simulink model "CPCS_nonlinear_modal"  (R2021a)
settings: Solver=VariableStepAuto  StartTime=0.0  StopTime=10.0  MaxStep=1e-4  RelTol=1e-3
values from neighbouring files (symbols this model uses):
  g = 9.81    [CPCS.m]
  M = m1+m2    (= 3.5)    [CPCS.m]
  m2 = .5    (= 0.5)    [CPCS.m]
  r = 0.5    [CPCS.m]
settings Model: Creator=raitaimoorali  LastModifiedBy=raitaimoorali

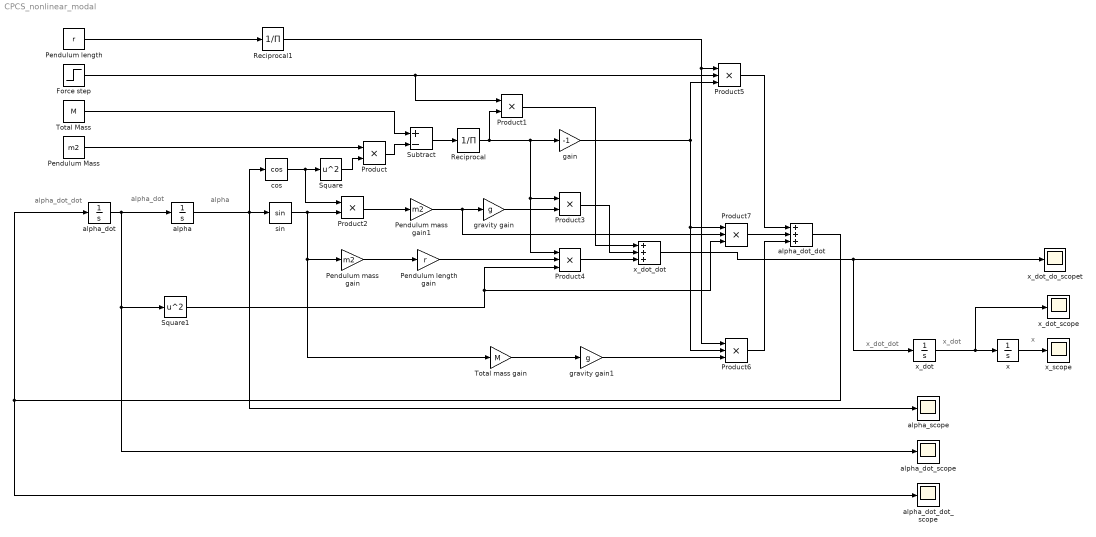
== system CPCS_nonlinear_modal ==
  note: x_dot_dot
  note: x_dot
  note: x
  note: alpha
  note: alpha_dot
  note: alpha_dot_dot
  Force step : Step  Time=0.01  SampleTime=0
  Pendulum Mass : Constant  Value=m2
  Pendulum length : Constant  Value=r
  Pendulum length gain : Gain  Gain=r
  Pendulum mass gain : Gain  Gain=m2
  Pendulum mass gain1 : Gain  Gain=m2
  Product{,1..3} (4 alike) : Product
  Product{4..7} (4 alike) : Product  Inputs=3
  Reciprocal : Product  Inputs=/
  Reciprocal1 : Product  Inputs=/
  Square : Math  Operator=square  SaturateOnIntegerOverflow=on
  Square1 : Math  Operator=square  SaturateOnIntegerOverflow=on
  Subtract : Sum  Inputs=+-
  Total Mass : Constant  Value=M
  Total mass gain : Gain  Gain=M
  alpha : Integrator
  alpha_dot : Integrator
  alpha_dot_dot : Sum  Inputs=+++
  alpha_dot_dot_scope : Scope
  alpha_dot_scope : Scope
  alpha_scope : Scope
  cos : Trigonometry  Operator=cos
  gain : Gain  Gain=-1
  gravity gain : Gain  Gain=g
  gravity gain1 : Gain  Gain=g
  sin : Trigonometry
  x : Integrator
  x_dot : Integrator
  x_dot_do_scopet : Scope
  x_dot_dot : Sum  Inputs=+++
  x_dot_scope : Scope
  x_scope : Scope
  wires:
  cos/1 -> Square/1, Product2/1
  Square/1 -> Product/2
  Pendulum Mass/1 -> Product/1
  Product/1 -> Subtract/2
  Total Mass/1 -> Subtract/1
  Force step/1 -> Product5/2, Product1/1
  Subtract/1 -> Reciprocal/1
  sin/1 -> Product2/2, Pendulum mass gain/1, Total mass gain/1
  Product2/1 -> Pendulum mass gain1/1
  gravity gain/1 -> Product3/2
  Pendulum mass gain/1 -> Pendulum length gain/1
  Pendulum length gain/1 -> Product4/2
  Square1/1 -> Product7/3, Product4/3
  Pendulum mass gain1/1 -> gravity gain/1, Product7/2
  Product1/1 -> x_dot_dot/1
  Product3/1 -> x_dot_dot/2
  Product4/1 -> x_dot_dot/3
  Reciprocal/1 -> Product1/2, gain/1, Product3/1, Product4/1
  Pendulum length/1 -> Reciprocal1/1
  gain/1 -> Product7/1, Product6/2, Product5/3
  Total mass gain/1 -> gravity gain1/1
  gravity gain1/1 -> Product6/3
  Reciprocal1/1 -> Product5/1, Product6/1
  Product5/1 -> alpha_dot_dot/1
  Product7/1 -> alpha_dot_dot/2
  Product6/1 -> alpha_dot_dot/3
  x/1 -> x_scope/1
  x_dot/1 -> x/1, x_dot_scope/1
  x_dot_dot/1 -> x_dot_do_scopet/1, x_dot/1
  alpha_dot_dot/1 -> alpha_dot_dot_scope/1, alpha_dot/1
  alpha/1 -> sin/1, cos/1, alpha_scope/1
  alpha_dot/1 -> alpha/1, Square1/1, alpha_dot_scope/1
